simulink model "PSI_Integration_to_Spherical_Angles"  (R2018b)
settings: Solver=VariableStepAuto  StartTime=0.0  StopTime=10.0  RelTol=1e-3
settings Model: Creator=thibault  LastModifiedBy=thibault

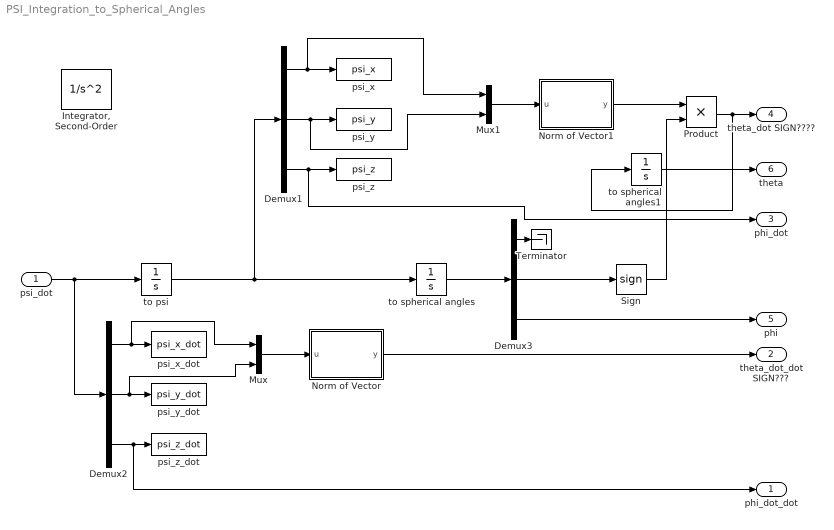
== system PSI_Integration_to_Spherical_Angles ==
  psi_dot : Inport
  Demux1 : Demux  Outputs=3
  Demux2 : Demux  Outputs=3
  Demux3 : Demux  Outputs=3
  "Integrator, Second-Order" : SecondOrderIntegrator
  Mux : Mux  Inputs=2
  Mux1 : Mux  Inputs=2
  Norm of Vector : MATLAB Function  TreatAsAtomicUnit=on
  Norm of Vector1 : MATLAB Function  TreatAsAtomicUnit=on
  Product : Product
  Sign : Signum
  Terminator : Terminator
  psi_x : ToWorkspace  VariableName=psi_x  SaveFormat=Timeseries  SampleTime=-1
  psi_x_dot : ToWorkspace  VariableName=psi_x_dot  SaveFormat=Timeseries  SampleTime=-1
  psi_y : ToWorkspace  VariableName=psi_y  SaveFormat=Timeseries  SampleTime=-1
  psi_y_dot : ToWorkspace  VariableName=psi_y_dot  SaveFormat=Timeseries  SampleTime=-1
  psi_z : ToWorkspace  VariableName=psi_z  SaveFormat=Timeseries  SampleTime=-1
  psi_z_dot : ToWorkspace  VariableName=psi_z_dot  SaveFormat=Timeseries  SampleTime=-1
  to psi : Integrator
  to spherical angles : Integrator  WrapState=on  WrappedStateUpperValue=2*pi  WrappedStateLowerValue=0  ZeroCross=off
  to spherical angles1 : Integrator  WrapState=on  WrappedStateLowerValue=0  ZeroCross=off
  phi_dot_dot : Outport
  theta_dot_dot SIGN??? : Outport  Port=2
  phi_dot : Outport  Port=3
  theta_dot SIGN???? : Outport  Port=4
  phi : Outport  Port=5
  theta : Outport  Port=6
  wires:
  to psi/1 -> Demux1/1, to spherical angles/1
  Demux2/1 -> Mux/1, psi_x_dot/1
  psi_dot/1 -> Demux2/1, to psi/1
  Demux2/2 -> psi_y_dot/1, Mux/2
  Demux2/3 -> psi_z_dot/1, phi_dot_dot/1
  Norm of Vector/1(y) -> theta_dot_dot SIGN???/1
  Mux/1 -> Norm of Vector/1(u)
  Demux1/2 -> Mux1/2, psi_y/1
  Demux1/3 -> phi_dot/1, psi_z/1
  Demux1/1 -> psi_x/1, Mux1/1
  Mux1/1 -> Norm of Vector1/1(u)
  Norm of Vector1/1(y) -> Product/1
  to spherical angles/1 -> Demux3/1
  Demux3/3 -> phi/1
  Demux3/1 -> Terminator/1
  Demux3/2 -> Sign/1
  Sign/1 -> Product/2
  Product/1 -> to spherical angles1/1, theta_dot SIGN????/1
  to spherical angles1/1 -> theta/1

== matlab function PSI_Integration_to_Spherical_Angles/Norm of Vector1 ==
  data: u input; y output
function y = norm_vector(u)

y = norm(u);
end

== matlab function PSI_Integration_to_Spherical_Angles/Norm of Vector ==
  data: u input; y output
function y = norm_vector(u)

y = norm(u);
end
